simulink model "PID_sim_6_25"  (R2018b)
settings: Solver=FixedStepAuto  StartTime=0.0  StopTime=10  FixedStep=0.05  RelTol=1e-3
settings Model: Creator=robolux  LastModifiedBy=robolux

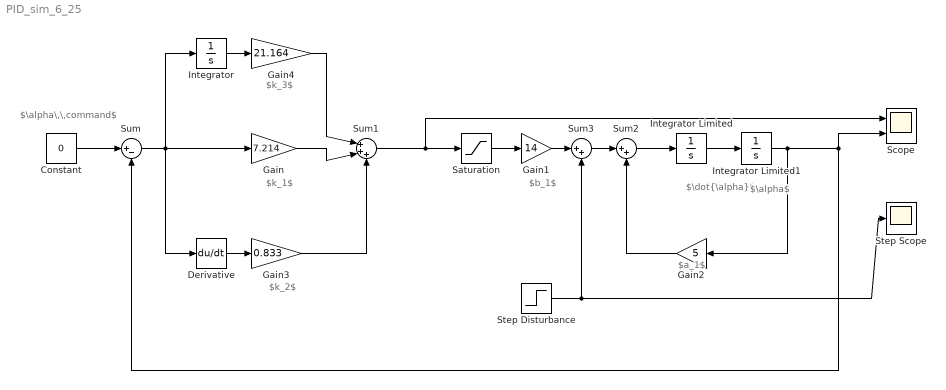
== system PID_sim_6_25 ==
  note: $\alpha\,\,command$
  note: $k_1$
  note: $k_2$
  note: $k_3$
  note: $b_1$
  note: $\dot{\alpha}$
  note: $\alpha$
  note: $a_1$
  Constant : Constant  Value=0
  Derivative : Derivative
  Gain : Gain  Gain=7.214
  Gain1 : Gain  Gain=14
  Gain2 : Gain  Gain=5
  Gain3 : Gain  Gain=0.833
  Gain4 : Gain  Gain=21.164
  Integrator : Integrator
  Integrator Limited : Integrator  InitialCondition=0.5  LimitOutput=on  UpperSaturationLimit=pi/6  LowerSaturationLimit=-pi/6
  Integrator Limited1 : Integrator  InitialCondition=0.1  LimitOutput=on  UpperSaturationLimit=pi/6  LowerSaturationLimit=-pi/6
  Saturation : Saturate  UpperLimit=pi/6  LowerLimit=-pi/6
  Scope : Scope  NumInputPorts=2
  Step Disturbance : Step  Time=4  After=6.25  SampleTime=0
  Step Scope : Scope
  Sum : Sum  Inputs=|+-
  Sum1 : Sum  Inputs=|+++
  Sum2 : Sum  Inputs=|++
  Sum3 : Sum  Inputs=|++
  wires:
  Integrator/1 -> Gain4/1
  Gain4/1 -> Sum1/1
  Gain1/1 -> Sum3/1
  Constant/1 -> Sum/1
  Integrator Limited/1 -> Integrator Limited1/1
  Integrator Limited1/1 -> Gain2/1, Sum/2, Scope/2
  Gain3/1 -> Sum1/3
  Step Disturbance/1 -> Step Scope/1, Sum3/2
  Sum3/1 -> Sum2/1
  Gain2/1 -> Sum2/2
  Sum2/1 -> Integrator Limited/1
  Derivative/1 -> Gain3/1
  Sum/1 -> Integrator/1, Derivative/1, Gain/1
  Gain/1 -> Sum1/2
  Saturation/1 -> Gain1/1
  Sum1/1 -> Scope/1, Saturation/1
